simulink model "GPCA_Extension"  (Simulink 7.9)
settings: Solver=ode45  StartTime=0.0  StopTime=inf  RelTol=1e-3
PreLoadFcn:
  | GPCA_Bus_Def
InitFcn:
  | script
undefined symbols (not defined in the file or in its folder): GOutputEvents, GProgrammedDoseRate, GProgrammedVTBI
libraries: simulink x6
(part 3 of 3)

== stateflow chart GPCA Software Controller/Alarming Component ==
  state AlarmingMachine
    state WRN [parallel]
      settings: executionOrder=5
      state HumidityCheck
      state BatteryChargingCheck
      state LowBatteryCheck
      state LoggingCheck
      state InfusionPausedDurationCheck
      state EndState
      state WNStart
        en: WnCond = 0;
      state LowReservoirCheck
      state VoltageCheck
      state FlowRateStabilityCheck
      state HoldOn
      state PumpTempCheck
      state EnvTempCheck
      state APErrCheck
      (junction 1019) -> (junction 1018)
      BatteryChargingCheck -> VoltageCheck [order 2] : [hardwareSenData.isBatteryUnableToCharge == 0]{clearWarning(21);}
      (junction 1020) -> (junction 1019)
      LowBatteryCheck -> BatteryChargingCheck [order 2] : [hardwareSenData.isBatteryLow ==0]{clearWarning(20);}
      LoggingCheck -> LowBatteryCheck [order 2] : [hardwareSenData.isLoggingFailed == 0]{clearWarning(19);}
      (junction 1035) -> LowReservoirCheck : {WnCond := 16; send(E_WarningAlarm, Controller);}
      LowReservoirCheck -> (junction 1036) [order 3] : [infuSenData.isReservoirLow > 0 && infusionInProgress > 0 ]
      (junction 1040) -> VoltageCheck : {WnCond := 21; send(E_WarningAlarm, Controller);}
      LowReservoirCheck -> (junction 1013) [order 1] : E_ResetThree
      InfusionPausedDurationCheck -> (junction 1014) [order 1] : E_ResetThree
      LowReservoirCheck -> InfusionPausedDurationCheck [order 2] : [infuSenData.isReservoirLow == 0 || infusionInProgress == 0 ]{clearWarning(17);}
      LoggingCheck -> (junction 1015) [order 1] : E_ResetThree
      LowBatteryCheck -> (junction 1017) [order 1] : E_ResetThree
      BatteryChargingCheck -> (junction 1018) [order 1] : E_ResetThree
      EndState -> WNStart : E_Clock{send(E_DoneThree, Controller);}
      (junction 1045) -> (junction 1043)
      VoltageCheck -> (junction 980) [order 3] : [hardwareSenData.isSupplyVoltageOutOfRange > 0]
      (default) -> WNStart
      WNStart -> HoldOn : E_ResetThree
      HoldOn -> FlowRateStabilityCheck : E_Clock{WnCond := 0;}
      (junction 1041) -> EnvTempCheck : {WnCond := 23; send(E_WarningAlarm, Controller);}
      AlarmingMachine.WRN.PumpTempCheck -> (junction 1041) [order 3] : [hardwareSenData.isPumpOverheated > 0]
      (junction 1038) -> LowBatteryCheck : {WnCond := 19; send(E_WarningAlarm, Controller);}
      VoltageCheck -> (junction 1019) [order 1] : E_ResetThree
      AlarmingMachine.WRN.PumpTempCheck -> (junction 1020) [order 1] : E_ResetThree
      (junction 1036) -> InfusionPausedDurationCheck : {WnCond := 17; send(E_WarningAlarm, Controller);}
      InfusionPausedDurationCheck -> LoggingCheck [order 2] : [infuSenData.isInfusionPausedLong == 0 || infusionInProgress == 0 || infusionPaused == 0]{clearWarning(18);}
      (junction 980) -> AlarmingMachine.WRN.PumpTempCheck : {WnCond := 22; send(E_WarningAlarm, Controller);}
      (junction 1044) -> APErrCheck : {WnCond := 25; send(E_WarningAlarm, Controller);}
      (junction 1003) -> WNStart : E_Clock{send(E_DoneThree, Controller);}
      BatteryChargingCheck -> (junction 1040) [order 3] : [hardwareSenData.isBatteryUnableToCharge > 0]
      (junction 1039) -> BatteryChargingCheck : {WnCond := 20; send(E_WarningAlarm, Controller);}
      LowBatteryCheck -> (junction 1039) [order 3] : [hardwareSenData.isBatteryLow > 0]
      FlowRateStabilityCheck -> (junction 1016) [order 1] : E_ResetThree
      FlowRateStabilityCheck -> LowReservoirCheck [order 2] : [infuSenData.isFlowRateNotStable == 0 || infusionInProgress == 0 || infusionPaused == 0]{clearWarning(16);}
      FlowRateStabilityCheck -> (junction 1035) [order 3] : [infuSenData.isFlowRateNotStable > 0 && infusionInProgress > 0 && infusionPaused == 0]
      (junction 1016) -> HoldOn
      (junction 1013) -> (junction 1016)
      (junction 1014) -> (junction 1013)
      (junction 1015) -> (junction 1014)
      (junction 1017) -> (junction 1015)
      (junction 1018) -> (junction 1017)
      InfusionPausedDurationCheck -> (junction 1037) [order 3] : [infuSenData.isInfusionPausedLong > 0 && infusionInProgress>0 && infusionPaused == 1]
      (junction 1037) -> LoggingCheck : {WnCond := 18; send(E_WarningAlarm, Controller);}
      LoggingCheck -> (junction 1038) [order 3] : [hardwareSenData.isLoggingFailed > 0]
      EnvTempCheck -> (junction 1043) [order 1] : E_ResetThree
      EnvTempCheck -> (junction 1042) [order 3] : [envSenData.isTemperatureOutOfRange > 0]
      (junction 1042) -> HumidityCheck : {WnCond := 24; send(E_WarningAlarm, Controller);}
      (junction 1043) -> (junction 1020)
      HumidityCheck -> (junction 1045) [order 1] : E_ResetThree
      HumidityCheck -> (junction 1044) [order 3] : [envSenData.isHumidityOutOfRange > 0]
      APErrCheck -> (junction 1003) [order 2] : [envSenData.isAirPressureOutOfRange ==0]{clearWarning(26);}
      APErrCheck -> (junction 1046) [order 1] : E_ResetThree
      HumidityCheck -> APErrCheck [order 2] : [envSenData.isHumidityOutOfRange == 0]{clearWarning(25);}
      (junction 1046) -> (junction 1045)
      VoltageCheck -> AlarmingMachine.WRN.PumpTempCheck [order 2] : [hardwareSenData.isSupplyVoltageOutOfRange == 0]{clearWarning(22);}
      AlarmingMachine.WRN.PumpTempCheck -> EnvTempCheck [order 2] : [hardwareSenData.isPumpOverheated == 0]{clearWarning(23);}
      EnvTempCheck -> HumidityCheck [order 2] : [envSenData.isTemperatureOutOfRange == 0]{clearWarning(24);}
      APErrCheck -> (junction 1047) [order 3] : [envSenData.isAirPressureOutOfRange > 0]
      (junction 1047) -> EndState : {WnCond := 26; send(E_WarningAlarm, Controller);}
    state Controller [parallel]
      settings: executionOrder=1
      state SinkTWOCheckOne
      state START
        en: initiate();
      state CheckLOne
        en:  initiate();
      state CheckWRN
      state SinkOne
      state SinkTWO
      state CheckLTwo
      CheckWRN -> CheckLOne [order 2] : E_DoneThree{send(E_ResetOne, LOne);}
      SinkOne -> CheckLOne : E_Restart{send(E_ResetOne, LOne);}
      CheckLOne -> SinkOne [order 1] : E_LevelOneAlarm{ErrCond:=LOneCond;}
      START -> CheckLOne : E_Restart{send(E_ResetOne, LOne);}
      (default) -> START
      CheckWRN -> CheckWRN [order 1] : E_WarningAlarm{ErrCond:=WnCond; E_Warning}
      CheckLTwo -> CheckWRN [order 3] : E_DoneTwo{send(E_ResetThree, WRN);}
      SinkTWOCheckOne -> SinkTWO [order 2] : E_DoneOne
      CheckLTwo -> SinkTWO [order 2] : E_LevelTwoAlarm{ErrCond:=LTwoCond;}
      SinkTWO -> SinkTWOCheckOne [order 3] : [LTwoCond>0]{send(E_ResetOne, LOne);}
      CheckLOne -> CheckLTwo [order 2] : E_DoneOne{send(E_ResetTwo, LTwo);}
      CheckLTwo -> CheckLOne [order 1] : E_Restart{send(E_ResetOne, LOne);}
      CheckWRN -> CheckLOne [order 3] : E_Restart{send(E_ResetOne, LOne);}
      SinkTWO -> CheckLOne [order 2] : E_Restart|E_AlarmClear{ErrCond := 0; send(E_ResetOne, LOne);}
      SinkTWO -> CheckLOne [order 1] : E_Clock[LTwoCond==0]{ErrCond := 0; send(E_ResetOne, LOne);}
      SinkTWOCheckOne -> CheckLOne [order 3] : E_Restart|E_AlarmClear{ErrCond := LOneCond; send(E_ResetOne, LOne);}
      SinkTWOCheckOne -> SinkOne [order 1] : E_LevelOneAlarm{ErrCond:=LOneCond;}
    state LTwo [parallel]
      settings: executionOrder=4
      state Hold
      state Sink24
        en: LTwoCond = 10;
        send(E_LevelTwoAlarm, Controller);
      state Sink26
        en: LTwoCond=12;
        send(E_LevelTwoAlarm, Controller);
      state RateOverPumpCapacityCheck
      state LowInfusionRateCheck
      state RateLessThanKVOCheck
      state Sink25
        en: LTwoCond = 11;
        send(E_LevelTwoAlarm, Controller);
      state OcculusionCheck
      state Sink23
        en: LTwoCond = 9;
        send(E_LevelTwoAlarm, Controller);
      state HighInfusionRateCheck
      state Normal
        en: LTwoCond =0;
      state DoorOpenCheck
      state Sink22
        en: LTwoCond = 8;
        send(E_LevelTwoAlarm, Controller);
      state ReservoirEmptyCheck
      state Sink21
        en: LTwoCond=7;
        send(E_LevelTwoAlarm, Controller);
      state InfusionPauseDurationCheck
      state Sink27
        en: LTwoCond=13;
        send(E_LevelTwoAlarm, Controller);
      state AirInLineCheck
      state Sink29
        en: LTwoCond=15;
        send(E_LevelTwoAlarm, Controller);
      state Sink28
        en: LTwoCond=14;
        send(E_LevelTwoAlarm, Controller);
      AirInLineCheck -> Sink29 [order 2] : [infuSenData.isAirInLineDetected > 0 && infusionInProgress > 0]
      InfusionPauseDurationCheck -> AirInLineCheck [order 3] : [infuSenData.isInfusionPausedTooLong == 0  || infusionInProgress == 0 || infusionPaused == 0]
      InfusionPauseDurationCheck -> Sink28 [order 2] : [infuSenData.isInfusionPausedTooLong > 0  && infusionInProgress > 0 && infusionPaused == 1]
      Sink29 -> (junction 995) [order 2] : [infuSenData.isAirInLineDetected == 0 || infusionInProgress == 0]
      Sink29 -> (junction 994) [order 1] : E_ResetTwo
      Sink28 -> (junction 996) [order 2] : [infuSenData.isInfusionPausedTooLong == 0  || infusionInProgress == 0 || infusionPaused == 0]
      Sink28 -> (junction 997) [order 1] : E_ResetTwo
      (junction 982) -> DoorOpenCheck
      (junction 995) -> (junction 996)
      AirInLineCheck -> (junction 983) [order 1] : E_ResetTwo
      InfusionPauseDurationCheck -> (junction 984) [order 1] : E_ResetTwo
      RateOverPumpCapacityCheck -> InfusionPauseDurationCheck [order 3] : [infuSenData.isFlowRateOverPumpCapacity == 0 || infusionInProgress == 0]
      Sink27 -> (junction 998) [order 2] : [infuSenData.isFlowRateOverPumpCapacity == 0 || infusionInProgress == 0]
      RateOverPumpCapacityCheck -> Sink27 [order 2] : [infuSenData.isFlowRateOverPumpCapacity > 0 && infusionInProgress > 0 ]
      RateOverPumpCapacityCheck -> (junction 1034) [order 1] : E_ResetTwo
      Sink27 -> (junction 999) [order 1] : E_ResetTwo
      RateLessThanKVOCheck -> RateOverPumpCapacityCheck [order 3] : [infuSenData.isInfusionRateLessThanKVO == 0 || infusionInProgress == 0]
      Sink26 -> (junction 1001) [order 1] : E_ResetTwo
      RateLessThanKVOCheck -> (junction 1033) [order 1] : E_ResetTwo
      RateLessThanKVOCheck -> Sink26 [order 2] : [infuSenData.isInfusionRateLessThanKVO > 0 && infusionInProgress > 0]
      Sink26 -> (junction 1000) [order 2] : [infuSenData.isInfusionRateLessThanKVO == 0 || infusionInProgress == 0]
      LowInfusionRateCheck -> RateLessThanKVOCheck [order 3] : [infuSenData.isInfusionRateTooLow == 0 || infusionInProgress == 0 || infusionPaused > 0]
      Sink25 -> (junction 1002) [order 2] : [infuSenData.isInfusionRateTooLow == 0 || infusionInProgress == 0 || infusionPaused > 0]
      LowInfusionRateCheck -> (junction 1032) [order 1] : E_ResetTwo
      LowInfusionRateCheck -> Sink25 [order 2] : [infuSenData.isInfusionRateTooLow > 0 && infusionInProgress > 0 && infusionPaused == 0]
      Sink25 -> (junction 991) [order 1] : E_ResetTwo
      HighInfusionRateCheck -> LowInfusionRateCheck [order 3] : [infuSenData.isInfusionRateTooHigh == 0 || infusionInProgress == 0 || infusionPaused > 0]
      HighInfusionRateCheck -> Sink24 [order 2] : [infuSenData.isInfusionRateTooHigh > 0 && infusionInProgress > 0 && infusionPaused == 0]
      OcculusionCheck -> HighInfusionRateCheck [order 3] : [infuSenData.isOcclusionDetected == 0 || infusionInProgress == 0]
      OcculusionCheck -> Sink23 [order 2] : [infuSenData.isOcclusionDetected > 0 && infusionInProgress > 0]
      Sink24 -> (junction 978) [order 1] : E_ResetTwo
      Sink24 -> (junction 979) [order 2] : [infuSenData.isInfusionRateTooHigh == 0 || infusionInProgress == 0 || infusionPaused > 0]
      Sink23 -> (junction 992) [order 2] : [infuSenData.isOcclusionDetected == 0 || infusionInProgress == 0]
      Sink23 -> (junction 993) [order 1] : E_ResetTwo
      ReservoirEmptyCheck -> OcculusionCheck [order 3] : [infuSenData.isReservoirEmpty == 0 || infusionInProgress == 0]
      ReservoirEmptyCheck -> Sink22 [order 2] : [infuSenData.isReservoirEmpty > 0 && infusionInProgress > 0]
      ReservoirEmptyCheck -> (junction 1029) [order 1] : E_ResetTwo
      HighInfusionRateCheck -> (junction 1031) [order 1] : E_ResetTwo
      OcculusionCheck -> (junction 1030) [order 1] : E_ResetTwo
      Sink22 -> (junction 988) [order 2] : [infuSenData.isReservoirEmpty == 0 || infusionInProgress == 0]
      Sink22 -> (junction 989) [order 1] : E_ResetTwo
      Sink21 -> (junction 986) [order 2] : [hardwareSenData.isReservoirDoorOpen == 0 || infusionInProgress == 0]
      Sink21 -> (junction 985) [order 1] : E_ResetTwo
      DoorOpenCheck -> Sink21 [order 2] : [hardwareSenData.isReservoirDoorOpen > 0 && infusionInProgress > 0]
      DoorOpenCheck -> ReservoirEmptyCheck [order 3] : [hardwareSenData.isReservoirDoorOpen == 0 || infusionInProgress == 0]
      DoorOpenCheck -> (junction 1028) [order 1] : E_ResetTwo
      (junction 994) -> (junction 997)
      (junction 979) -> (junction 992)
      Hold -> DoorOpenCheck : E_Clock{LTwoCond=0;}
      (junction 978) -> (junction 993)
      (junction 997) -> (junction 999)
      (default) -> AlarmingMachine.LTwo.Normal
      AlarmingMachine.LTwo.Normal -> Hold : E_ResetTwo
      (junction 1028) -> Hold
      (junction 1030) -> (junction 1029)
      (junction 1031) -> (junction 1030)
      (junction 1029) -> (junction 1028)
      (junction 1034) -> (junction 1033)
      (junction 1033) -> (junction 1032)
      (junction 1032) -> (junction 1031)
      (junction 996) -> (junction 998)
      (junction 983) -> (junction 984)
      (junction 984) -> (junction 1034)
      (junction 1002) -> (junction 979)
      (junction 991) -> (junction 978)
      (junction 992) -> (junction 988)
      (junction 993) -> (junction 989)
      (junction 988) -> (junction 986)
      (junction 989) -> (junction 985)
      (junction 990) -> DoorOpenCheck : E_Clock
      (junction 986) -> (junction 990)
      (junction 985) -> (junction 982)
      (junction 1007) -> AlarmingMachine.LTwo.Normal : {send(E_DoneTwo, Controller);}
      AirInLineCheck -> (junction 1007) [order 3] : [infuSenData.isAirInLineDetected == 0 || infusionInProgress == 0]
      (junction 998) -> (junction 1000)
      (junction 999) -> (junction 1001)
      (junction 1000) -> (junction 1002)
      (junction 1001) -> (junction 991)
    state LOne [parallel]
      settings: executionOrder=3
      state HOLD
      state WatchdogCheck
      state MemoryCheck
      state CPUCheck
      state RTCCheck
      state Normal
      state PumpTempCheck
      state L1Sink
      state BatteryDepletionCheck
      (junction 1024) -> (junction 1022)
      WatchdogCheck -> L1Sink [order 2] : [hardwareSenData.isWatchDogInterruptDetected > 0]{LOneCond:=6; send(E_LevelOneAlarm, Controller);}
      AlarmingMachine.LOne.PumpTempCheck -> WatchdogCheck [order 3] : [hardwareSenData.isPumpTooHot == 0]
      AlarmingMachine.LOne.Normal -> HOLD : E_ResetOne
      WatchdogCheck -> (junction 1027) [order 3] : [hardwareSenData.isWatchDogInterruptDetected==0]{send(E_DoneOne, Controller);}
      WatchdogCheck -> (junction 1008) [order 1] : E_ResetOne
      (default) -> AlarmingMachine.LOne.Normal
      L1Sink -> HOLD : E_ResetOne
      AlarmingMachine.LOne.PumpTempCheck -> L1Sink [order 2] : [hardwareSenData.isPumpTooHot >0]{LOneCond:=5; send(E_LevelOneAlarm, Controller);}
      MemoryCheck -> AlarmingMachine.LOne.PumpTempCheck [order 3] : [hardwareSenData.isMemoryCorrupted == 0]
      MemoryCheck -> L1Sink [order 2] : [hardwareSenData.isMemoryCorrupted > 0]{LOneCond:=4; send(E_LevelOneAlarm, Controller);}
      CPUCheck -> MemoryCheck [order 3] : [hardwareSenData.isCPUInError == 0]
      CPUCheck -> L1Sink [order 2] : [hardwareSenData.isCPUInError > 0]{LOneCond := 3; send(E_LevelOneAlarm, Controller);}
      RTCCheck -> CPUCheck [order 3] : [hardwareSenData.isRTCInError > 0 == 0]
      RTCCheck -> L1Sink [order 2] : [hardwareSenData.isRTCInError > 0> 0]{LOneCond:=2; send(E_LevelOneAlarm, Controller);}
      BatteryDepletionCheck -> RTCCheck [order 3] : [hardwareSenData.isBatteryDepleted == 0]
      BatteryDepletionCheck -> L1Sink [order 2] : [hardwareSenData.isBatteryDepleted > 0]{LOneCond:=1; send(E_LevelOneAlarm, Controller);}
      MemoryCheck -> (junction 1025) [order 1] : E_ResetOne
      AlarmingMachine.LOne.PumpTempCheck -> (junction 1026) [order 1] : E_ResetOne
      CPUCheck -> (junction 1024) [order 1] : E_ResetOne
      RTCCheck -> (junction 1022) [order 1] : E_ResetOne
      BatteryDepletionCheck -> (junction 1021) [order 1] : E_ResetOne
      (junction 1021) -> HOLD
      HOLD -> BatteryDepletionCheck : E_Clock{LOneCond=0;}
      (junction 1008) -> (junction 1026)
      (junction 1027) -> AlarmingMachine.LOne.Normal : E_Clock
      (junction 1026) -> (junction 1025)
      (junction 1022) -> (junction 1021)
      (junction 1025) -> (junction 1024)
    state CheckReady [parallel]
      settings: executionOrder=2
      state Normal
      state s1
      state Checking
        en: temp := isPumpReady();
      state s2
      s2 -> AlarmingMachine.CheckReady.Normal [order 3] : E_Restart
      s2 -> s2 [order 2] : E_Clock{E_NotReady}
      s1 -> AlarmingMachine.CheckReady.Normal [order 4] : E_Restart
      s1 -> s1 [order 1] : E_Clock[infusionInProgress == 0]{E_Ready}
      Checking -> AlarmingMachine.CheckReady.Normal [order 1] : E_Restart
      s2 -> Checking [order 1] : E_RequestToStart
      s1 -> AlarmingMachine.CheckReady.Normal [order 2] : E_Clock[infusionInProgress == 1]
      s1 -> Checking [order 3] : E_RequestToStart
      (default) -> AlarmingMachine.CheckReady.Normal
      AlarmingMachine.CheckReady.Normal -> Checking : E_RequestToStart
      Checking -> s2 [order 3] : [temp == 0]
      Checking -> s1 [order 2] : [temp > 0]
    (default) -> Controller
  state x = clearWarning(cond) [function]
    (junction 1006) -> (junction 1005) [order 1] : [ErrCond != cond]{x:=0;}
    (junction 1006) -> (junction 1004) [order 2] : [ErrCond == cond]{ml.GAlrmMsg = MSG_BLANK; ErrCond := 0;}
    (default) -> (junction 1006)
  state x = isPumpReady [function]
    (junction 987) -> (junction 1009) [order 1] : [infuSenData.isReservoirEmpty > 0]{ x := 0;}
    (junction 981) -> (junction 1011) [order 1] : [hardwareSenData.isReservoirDoorOpen > 0] {x := 0;}
    (junction 987) -> (junction 981) [order 2] : [infuSenData.isReservoirEmpty == 0]
    (default) -> (junction 987)
    (junction 981) -> (junction 1010) [order 2] : [hardwareSenData.isReservoirDoorOpen == 0]
    (junction 1010) -> (junction 1023) [order 1] : [infuSenData.isFlowRateOverPumpCapacity > 0]{x := 0;}
    (junction 1010) -> (junction 1012) [order 2] : [infuSenData.isFlowRateOverPumpCapacity == 0]{x := 1;}
  state x = initiate [function]
    (default) -> (junction 977) : {LOneCond := 0; LTwoCond := 0; WnCond := 0; ErrCond := 0; x:=0;}
  (default) -> AlarmingMachine
  data: cond function_input uint32; x function_output uint32; x function_output uint32; x function_output uint32; ClearCond input int8; infusionInProgress input uint32; ErrCond output double; infusionPaused input double; envSenData input Bus: EnvironmentSensorSignals size=1; LOneCond local uint32; LTwoCond local uint32; WnCond local uint32; MSG_BLANK constant uint32 =30; hardwareSenData input Bus: HardwareSensorSignals size=1; infuSenData input Bus: InfusionSensorSignals size=1; temp local boolean
  events: E_Alarm output EITHER_EDGE_EVENT; E_Restart input RISING_EDGE_EVENT; E_AlarmClear input RISING_EDGE_EVENT; E_Warning output EITHER_EDGE_EVENT; E_LevelOneAlarm local EITHER_EDGE_EVENT; E_LevelTwoAlarm local EITHER_EDGE_EVENT; E_LevelOneClear local EITHER_EDGE_EVENT; E_ResetOne local EITHER_EDGE_EVENT; E_DoneOne local EITHER_EDGE_EVENT; E_DoneThree local EITHER_EDGE_EVENT; E_DoneTwo local EITHER_EDGE_EVENT; E_ResetTwo local EITHER_EDGE_EVENT; E_ResetThree local EITHER_EDGE_EVENT; E_WarningAlarm local EITHER_EDGE_EVENT; E_RequestToStart input EITHER_EDGE_EVENT; E_Clock input RISING_EDGE_EVENT; E_Ready output EITHER_EDGE_EVENT; E_NotReady output EITHER_EDGE_EVENT

== matlab function GPCA Software Controller/D2BC ==
  data: u input double; y output double
function y = d_to_b(u)
% This block supports the Embedded MATLAB subset.
% See the help menu for details. 

y = false;

if (u == 0)
    y = false;
else 
     y = true;
end;
